simulink model "sf_pw_ifelseif_"  (Simulink 7.4)
settings: Solver=FixedStepDiscrete  StartTime=0.0  StopTime=10.0  RelTol=1e-3
settings Model: Creator=vreddy  LastModifiedBy=rcobbe
settings ConfigSet: Description=Default Configuration
settings OptimizationCC: InlineParams=on  InlineInvariantSignals=on  StateBitsets=on  DataBitsets=on  UseTempVars=on  ZeroExternalMemoryAtStartup=off  ZeroInternalMemoryAtStartup=off  NoFixptDivByZeroProtection=on  EfficientFloat2IntCast=on  OptimizeModelRefInitCode=on  LifeSpan=1
settings DebuggingCC: SignalInfNanChecking=warning  SaveWithParameterizedLinksMsg=none
settings RTWCC: SystemTargetFile=ert.tlc  TemplateMakefile=ert_default_tmf  Description=Real-Time Workshop Embedded Coder (no auto configuration)  ProcessScript=ert_make_rtw_hook
settings CodeAppCC: IgnoreCustomStorageClasses=off
settings ERTTargetCC: TargetFcnLib=ansi_tfl_tmw.mat  MultiwordLength=2048  GenerateSampleERTMain=on  InlinedParameterPlacement=NonHierarchical  ERTCustomFileTemplate=example_file_process.tlc  ConvertIfToSwitch=off

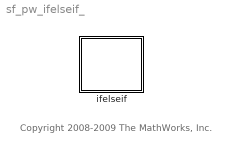
== system sf_pw_ifelseif_ ==
  note: Copyright 2008-2009 The MathWorks, Inc.
  ifelseif : Stateflow chart

== stateflow chart ifelseif ==
  (default) -> (junction 3) : /*comment*/
  (junction 3) -> (junction 5) [order 2]
  (junction 3) -> (junction 6) [order 1] : [condition1]
  (junction 6) -> (junction 7) : {action1}
  (junction 5) -> (junction 8) [order 1] : [condition2]
  (junction 8) -> (junction 9) : {action2}
  (junction 7) -> (junction 9)
  (junction 9) -> (junction 4)
  (junction 5) -> (junction 4) [order 2]
  (junction 4) -> (junction 10)
